simulink model "DC_Motor"  (R2015a)
settings: Solver=ode45  StartTime=0.0  StopTime=10.0  RelTol=1e-3
settings Model: Creator=Kunal  LastModifiedBy=Kunal

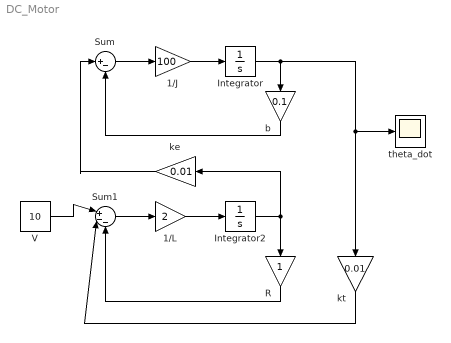
== system DC_Motor ==
  1/J : Gain  Gain=100
  1/L : Gain  Gain=2
  Integrator : Integrator
  Integrator2 : Integrator
  R : Gain
  Sum : Sum  Inputs=|+-
  Sum1 : Sum  Inputs=|+--
  V : Constant  Value=10
  b : Gain  Gain=0.1
  ke : Gain  Gain=0.01
  kt : Gain  Gain=0.01
  theta_dot : Scope
      settings: YMin=-0.2  YMax=1.2  MaxDataPoints=5000000
  wires:
  Integrator/1 -> theta_dot/1, kt/1, b/1
  b/1 -> Sum/2
  Sum/1 -> 1/J/1
  1/J/1 -> Integrator/1
  Integrator2/1 -> ke/1, R/1
  R/1 -> Sum1/3
  Sum1/1 -> 1/L/1
  1/L/1 -> Integrator2/1
  kt/1 -> Sum1/2
  ke/1 -> Sum/1
  V/1 -> Sum1/1
